simulink model "simulink1"  (R2017a)
settings: Solver=VariableStepAuto  StartTime=0.0  StopTime=10.0  RelTol=1e-3
values from neighbouring files (symbols this model uses):
  param = zeros(2,1)    [complete_parameter_estimation_script.m]    (also in parameter_estimation_script.m)
settings Model: Creator=asus  LastModifiedBy=asus

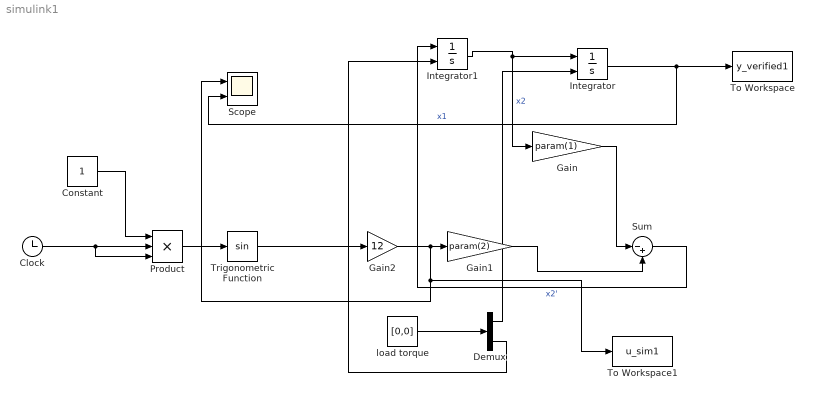
== system simulink1 ==
  Clock : Clock
  Constant : Constant
  Demux : Demux  Outputs=2
  Gain : Gain  Gain=param(1)
  Gain1 : Gain  Gain=param(2)
  Gain2 : Gain  Gain=12
  Integrator : Integrator  InitialConditionSource=external
  Integrator1 : Integrator  InitialConditionSource=external
  Product : Product  Inputs=3
  Scope : Scope  NumInputPorts=2
  Sum : Sum  Inputs=|-+
  To Workspace : ToWorkspace  VariableName=y_verified1  SaveFormat=Timeseries  SampleTime=-1
  To Workspace1 : ToWorkspace  VariableName=u_sim1  SaveFormat=Timeseries  SampleTime=-1
  Trigonometric Function : Trigonometry
  load torque : Constant  Value=[0,0]
  wires:
  Integrator/1 -> Scope/2, To Workspace/1  "x1"
  Sum/1 -> Integrator1/1  "x2'"
  Gain2/1 -> Scope/1, To Workspace1/1, Gain1/1
  Gain/1 -> Sum/1
  Gain1/1 -> Sum/2
  Integrator1/1 -> Integrator/1, Gain/1  "x2"
  Demux/2 -> Integrator1/2
  load torque/1 -> Demux/1
  Demux/1 -> Integrator/2
  Trigonometric Function/1 -> Gain2/1
  Product/1 -> Trigonometric Function/1
  Constant/1 -> Product/1
  Clock/1 -> Product/3, Product/2
